simulink library "Yaw_Gearbox_Lib_org"  (Simulink 10.0)
settings: Solver=ode45  StartTime=0.0  StopTime=10.0  RelTol=1e-3  EnableMultiTasking=on
undefined symbols (not defined in the file): WT_Params
libraries: fl_lib x7, sdl_lib x4
Description:
  | Copyright 2009-2017 The MathWorks, Inc. MathWorks, Inc.
settings Model: Creator=smiller  LastModifiedBy=annonymous

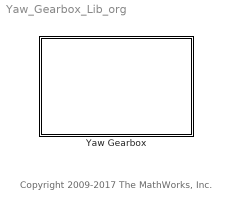
== system Yaw_Gearbox_Lib_org ==
  note: Copyright 2009-2017 The MathWorks, Inc.
  Yaw Gearbox : Subsystem
      mask Display: image(imread('Yaw_Gearbox_IMAGE.jpg'));

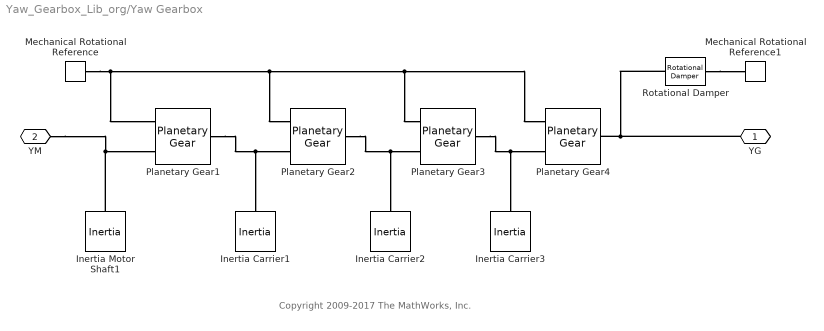
== system Yaw_Gearbox_Lib_org/Yaw Gearbox ==
  note: Copyright 2009-2017 The MathWorks, Inc.
  Inertia Carrier1 : fl_lib/Mechanical/Rotational Elements/Inertia  inertia=WT_Params.Yaw_Actuator.inertia_carrier kg*m^2  w_specify=on  w_priority=High  w=0 rad/s  w_nominal_specify=off  w_nominal_unit=rad/s  w_nominal_value=1  t_specify=off  t_priority=High  t=0 N*m  t_nominal_specify=off  t_nominal_unit=N*m  t_nominal_value=1
  Inertia Carrier2 : fl_lib/Mechanical/Rotational Elements/Inertia  inertia=WT_Params.Yaw_Actuator.inertia_carrier kg*m^2  w_specify=on  w_priority=High  w=0 rad/s  w_nominal_specify=off  w_nominal_unit=rad/s  w_nominal_value=1  t_specify=off  t_priority=High  t=0 N*m  t_nominal_specify=off  t_nominal_unit=N*m  t_nominal_value=1
  Inertia Carrier3 : fl_lib/Mechanical/Rotational Elements/Inertia  inertia=WT_Params.Yaw_Actuator.inertia_carrier kg*m^2  w_specify=on  w_priority=High  w=0 rad/s  w_nominal_specify=off  w_nominal_unit=rad/s  w_nominal_value=1  t_specify=off  t_priority=High  t=0 N*m  t_nominal_specify=off  t_nominal_unit=N*m  t_nominal_value=1
  Inertia Motor Shaft1 : fl_lib/Mechanical/Rotational Elements/Inertia  inertia=WT_Params.Yaw_Actuator.inertia_motor_shaft kg*m^2  w_specify=on  w_priority=High  w=0 rad/s  w_nominal_specify=off  w_nominal_unit=rad/s  w_nominal_value=1  t_specify=off  t_priority=High  t=0 N*m  t_nominal_specify=off  t_nominal_unit=N*m  t_nominal_value=1
  Mechanical Rotational Reference : fl_lib/Mechanical/Rotational Elements/Mechanical Rotational Reference
  Mechanical Rotational Reference1 : fl_lib/Mechanical/Rotational Elements/Mechanical Rotational Reference
  Planetary Gear1 : sdl_lib/Gears/Planetary Gear  rs_ratio=WT_Params.Yaw_Actuator.p_gear_rato_step_1-1  friction_model=1  efficiency=[ 0.96 0.98 ]  mu_visc=[ 0 0 ] N*m/(rad/s)  pwr_thr=[ 0.001 0.001 ] W  planet_inertia=0 kg*m^2  temperature_TLU=[ 280 300 320 ] K  efficiency_sp_TLU=[ 0.95 0.9 0.85 ]  efficiency_rp_TLU=[ 0.95 0.9 0.85 ]  thermal_mass=50 J/K  T_init=300 K
      settings: SourceProductName=Simscape Driveline  SourceProductBaseCode=LD
  Planetary Gear2 : sdl_lib/Gears/Planetary Gear  rs_ratio=WT_Params.Yaw_Actuator.p_gear_rato_step_2-1  friction_model=1  efficiency=[ 0.96 0.98 ]  mu_visc=[ 0 0 ] N*m/(rad/s)  pwr_thr=[ 0.001 0.001 ] W  planet_inertia=0 kg*m^2  temperature_TLU=[ 280 300 320 ] K  efficiency_sp_TLU=[ 0.95 0.9 0.85 ]  efficiency_rp_TLU=[ 0.95 0.9 0.85 ]  thermal_mass=50 J/K  T_init=300 K
      settings: SourceProductName=Simscape Driveline  SourceProductBaseCode=LD
  Planetary Gear3 : sdl_lib/Gears/Planetary Gear  rs_ratio=WT_Params.Yaw_Actuator.p_gear_rato_step_3-1  friction_model=1  efficiency=[ 0.96 0.98 ]  mu_visc=[ 0 0 ] N*m/(rad/s)  pwr_thr=[ 0.001 0.001 ] W  planet_inertia=0 kg*m^2  temperature_TLU=[ 280 300 320 ] K  efficiency_sp_TLU=[ 0.95 0.9 0.85 ]  efficiency_rp_TLU=[ 0.95 0.9 0.85 ]  thermal_mass=50 J/K  T_init=300 K
      settings: SourceProductName=Simscape Driveline  SourceProductBaseCode=LD
  Planetary Gear4 : sdl_lib/Gears/Planetary Gear  rs_ratio=WT_Params.Yaw_Actuator.p_gear_rato_step_4-1  friction_model=1  efficiency=[ 0.96 0.98 ]  mu_visc=[ 0 0 ] N*m/(rad/s)  pwr_thr=[ 0.001 0.001 ] W  planet_inertia=0 kg*m^2  temperature_TLU=[ 280 300 320 ] K  efficiency_sp_TLU=[ 0.95 0.9 0.85 ]  efficiency_rp_TLU=[ 0.95 0.9 0.85 ]  thermal_mass=50 J/K  T_init=300 K
      settings: SourceProductName=Simscape Driveline  SourceProductBaseCode=LD
  Rotational Damper : fl_lib/Mechanical/Rotational Elements/Rotational Damper  D=WT_Params.Yaw_Actuator.damping N*m/(rad/s)  w_specify=off  w_priority=High  w=0 rad/s  w_nominal_specify=off  w_nominal_unit=rad/s  w_nominal_value=1  t_specify=off  t_priority=High  t=0 N*m  t_nominal_specify=off  t_nominal_unit=N*m  t_nominal_value=1
  YG : PMIOPort  Side=Right
  YM : PMIOPort  Port=2  Side=Left
  connections:
  Planetary Gear1/LConn1 -- Planetary Gear2/RConn2 -- Inertia Carrier1/LConn1
  Planetary Gear2/LConn1 -- Planetary Gear3/RConn2 -- Inertia Carrier2/LConn1
  Planetary Gear3/LConn1 -- Planetary Gear4/RConn2 -- Inertia Carrier3/LConn1
  Mechanical Rotational Reference/LConn1 -- Planetary Gear1/RConn1 -- Planetary Gear2/RConn1 -- Planetary Gear3/RConn1 -- Planetary Gear4/RConn1
  Inertia Motor Shaft1/LConn1 -- Planetary Gear1/RConn2 -- YM/RConn1
  Rotational Damper/LConn1 -- YG/RConn1 -- Planetary Gear4/LConn1
  Rotational Damper/RConn1 -- Mechanical Rotational Reference1/LConn1
